simulink model "UNIFIER_dyn"  (R2023b)
settings: Solver=VariableStepAuto  StartTime=0.0  StopTime=10  RelTol=1e-3
InitFcn:
  | UNIFIER_LOAD
values from neighbouring files (symbols this model uses):
  b = 20.11467    [UNIFIER_LOAD.m]    (also in UNIFIER_LOAD.mat; UNIFIER_LOAD_ROM.m; UNIFIER_LOAD_ROM.mat)
  c = 1.43676    [UNIFIER_LOAD.m]    (also in UNIFIER_LOAD.mat; UNIFIER_LOAD_ROM.m; UNIFIER_LOAD_ROM.mat)
  dp_DEP =     [UNIFIER_LOAD.mat]    (also in UNIFIER_LOAD_ROM.mat)
  dp_FUSE_FIN =     [UNIFIER_LOAD.mat]
  dp_HTU =     [UNIFIER_LOAD.mat]    (also in UNIFIER_LOAD_ROM.mat)
  dp_VTAIL =     [UNIFIER_LOAD.mat]
  dp_VTAIL_INDUCED =     [UNIFIER_LOAD.mat]
  dp_WING_root =     [UNIFIER_LOAD.mat]
  dp_WING_tip =     [UNIFIER_LOAD.mat]
  I = [23600,     -0,  -1740 ... (first row only)    [UNIFIER_LOAD.m]    (also in UNIFIER_LOAD.mat = [23600  0  -1740; 0  89800  0; -1740  0  102000]; UNIFIER_LOAD_ROM.m = [23600,     -0,   -1740; UNIFIER_LOAD_ROM.mat = [23600  0  -1740; 0  89800  0; -1740  0  102000])
  m = 7057    [UNIFIER_LOAD.m]    (also in UNIFIER_LOAD.mat; UNIFIER_LOAD_ROM.m; UNIFIER_LOAD_ROM.mat)
  S = 29.98388    [UNIFIER_LOAD.m]    (also in UNIFIER_LOAD.mat; UNIFIER_LOAD_ROM.m; UNIFIER_LOAD_ROM.mat)
  vtail_nodes = [dp_VTAIL.Xs_LE;     dp_VTAIL.Ys_LE;     dp_VTAIL.Zs_LE]    [UNIFIER_LOAD.m]    (also in UNIFIER_LOAD.mat = [-16.4894695282 -2.83441376686 -2.73765826225 -16.1370849609)
  wing_nodes = [fliplr(dp_WING_tip.LE_Xs),fliplr(dp_WING_root.LE_Xs),dp_WING_root.LE_Xs,dp_WING_tip.LE_Xs;     fliplr(-dp_WING_tip.LE_Ys),fliplr(-dp_WING_root.LE_Ys),dp_WING_root.LE_Ys,dp_WING_tip.LE_Ys;     fliplr(dp_WING_tip.LE_Zs),fliplr(dp_WING_root.LE_Zs),dp_WING_root.LE_Zs,dp_WING_tip.LE_Zs]    [UNIFIER_LOAD.m]    (also in UNIFIER_LOAD.mat = [-7.70795631409 -9.67500019073 -0.98178178072 -7.66801691055)
  X = target.X    [OptimalTracking_UNIFIER_obj.m]
  xyz_cg = [-8.09,0,-0.2]    [UNIFIER_LOAD.m]    (also in UNIFIER_LOAD.mat = [-8.09 0 -0.2]; UNIFIER_LOAD_ROM.m; UNIFIER_LOAD_ROM.mat = [-8.09 0 -0.2])
  xyz_DEP = [ -6.9629998	-6.9210000	-6.8660002	-6.8099999	-6.7540002	-6.6999998	-6.6999998	-6.7540002	-6.8099999	-6.8660002	-6.9210000	-6.9629998 ... (first row only)    [UNIFIER_LOAD.m]    (also in UNIFIER_LOAD.mat = [-6.9629998 -10.05 -0.90899998 -6.921 -8.4499998 -0.792 -6.8; UNIFIER_LOAD_ROM.m; UNIFIER_LOAD_ROM.mat = [-6.9629998 -10.05 -0.90899998 -6.921 -8.4499998 -0.792 -6.8)
undefined symbols (not defined in the file or in its folder): OBM, U, unifier_obm
libraries: sharedutil x7, aerolibtransform2 x4, sharedtransform x2, aerolibatmos2 x1, matrix_library x1, shared6dofsys x1, shared6dof x1, simulink x1
(part 1 of 3)
settings Model: SimulationMode=rapid-accelerator  Creator=Reggie Johanes  LastModifiedBy=Reggie Johanes
settings DebuggingCC: ParameterPrecisionLossMsg=none

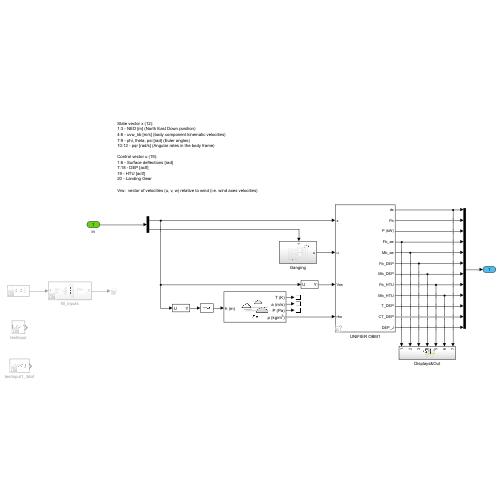
[thumbnail: Simulink's stored preview of the top-level diagram]
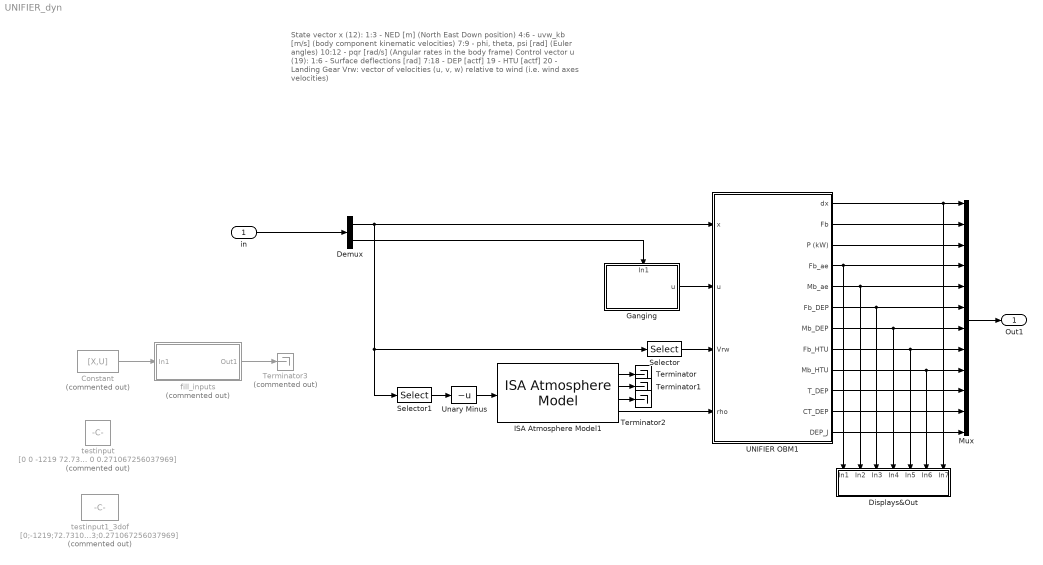
== system UNIFIER_dyn ==
  note: State vector x (12):
      | 1:3 - NED [m] (North East Down position)
      | 4:6 - uvw_kb [m/s] (body component kinematic velocities)
      | 7:9 - phi, theta, psi [rad] (Euler angles)
      | 10:12 - pqr [rad/s] (Angular rates in the body frame)
      |
      | Control vector u (19):
      | 1:6 - Surface deflections [rad]
      | 7:18 - DEP [actf]
      | 19 - HTU [actf]
      | 20 - Landing Gear
      |
      | Vrw:  vector of velocities (u, v, w) relative to wind (i.e. wind axes velocities)
  in : Inport
  Constant : Constant  Commented=on  Value=[X,U]
  Demux : Demux  Outputs=[12,7]
  Displays&Out : Subsystem
  Ganging : Subsystem
      settings: PortSchema="{\"entries\":[{\"content\":{\"sides\":[{\"content\":{},\"type\":\"ConnectorPlacement.EquallySpacedRectSide\",\"uuid\":\"ab643a29-1b81-4d77-b01e-60bacc52a34e\"},{\"content\":{\"connectorIds\":[\"Out1\"],\"side\":\"RIGHT\"},\"type\":\"ConnectorPlacement.EquallySpacedRectSide\",\"uuid\":\"168c35b5-3601-4e59-863f-07713e2152c6\"},{\"content\":{\"connectorIds\":[\"In1\"],\"side\":\"TOP\"},\"type\":\"ConnectorPlacement.EquallySpacedRectSide\",\"uuid\":\"1288536c-167d-4f59-8222-829bbd711e20\"}]},\"type\":\"ConnectorPlacement.EquallySpacedConnector\",\"uuid\":\"db641389-38bb-4549-8fb7-216d33e1be74\"}],\"packageUris\":[\"http://schema.mathworks.com/mf0/Connector/R2020b\"],\"version\":\"1.0\"}"
  ISA Atmosphere Model1 : aerolibatmos2/ISA Atmosphere Model  useExtended=off  action=Warning  custom=off  viscosityOut=off  g=9.80665  gamma=1.4  R=287.0531  L=0.0065  h_trop=11000  h_strat=20000  rho0=1.225  P0=101325  T0=288.15  h0=0
  Mux : Mux  Inputs=12
  Selector : Selector  InputPortWidth=12  IndexOptions=Index vector (dialog)  Indices=[4 5 6]  OutputSizes=1
  Selector1 : Selector  InputPortWidth=12  IndexOptions=Index vector (dialog)  Indices=[3]  OutputSizes=1
  Terminator : Terminator
  Terminator1 : Terminator
  Terminator2 : Terminator
  Terminator3 : Terminator  Commented=on
  UNIFIER OBM1 : Subsystem  AncestorBlock=unifier_obm/OBM
  Unary Minus : UnaryMinus
  fill_inputs : Subsystem  Commented=on
  testinput : Constant  Commented=on  Value=|
      | [0
      | 0
      | -1219
      | 72.7310470326144
      | 0
      | 1.14230710451874
      | 0
      | 0.0157060522826662
      | 0
      | 0
      | 0
      | 0
      | 0
      | 0
      | -0.0152983206921004
      | 0
      | 0.306978739246813
      | 0
      | 0.271067256037969]
  testinput1_3dof : Constant  Commented=on  Value=[0;-1219;72.731047032614440;1.142307104518741;0.015706052282666;0;-0.015298320692100;0;0.306978739246813;0.271067256037969]
  Out1 : Outport
  wires:
  Demux/1 -> Selector/1, Selector1/1, UNIFIER OBM1/1(x)
  Selector1/1 -> Unary Minus/1
  Unary Minus/1 -> ISA Atmosphere Model1/1
  ISA Atmosphere Model1/1 -> Terminator/1
  ISA Atmosphere Model1/2 -> Terminator1/1
  ISA Atmosphere Model1/3 -> Terminator2/1
  ISA Atmosphere Model1/4 -> UNIFIER OBM1/4(rho)
  Selector/1 -> UNIFIER OBM1/3(Vrw)
  Ganging/1(u) -> UNIFIER OBM1/2(u)
  Demux/2 -> Ganging/1(In1)
  UNIFIER OBM1/6(Fb_DEP) -> Mux/6, Displays&Out/3(In3)
  UNIFIER OBM1/4(Fb_ae) -> Mux/4, Displays&Out/1(In1)
  UNIFIER OBM1/7(Mb_DEP) -> Mux/7, Displays&Out/4(In4)
  UNIFIER OBM1/8(Fb_HTU) -> Mux/8, Displays&Out/5(In5)
  UNIFIER OBM1/11(CT_DEP) -> Mux/11
  UNIFIER OBM1/2(Fb) -> Mux/2
  UNIFIER OBM1/9(Mb_HTU) -> Mux/9, Displays&Out/6(In6)
  UNIFIER OBM1/3(P (kW)) -> Mux/3
  UNIFIER OBM1/10(T_DEP) -> Mux/10
  UNIFIER OBM1/1(dx) -> Displays&Out/7(In7), Mux/1
  Mux/1 -> Out1/1
  UNIFIER OBM1/12(DEP_J) -> Mux/12
  UNIFIER OBM1/5(Mb_ae) -> Mux/5, Displays&Out/2(In2)
  in/1 -> Demux/1
  Constant/1 -> fill_inputs/1(In1)
  fill_inputs/1(Out1) -> Terminator3/1

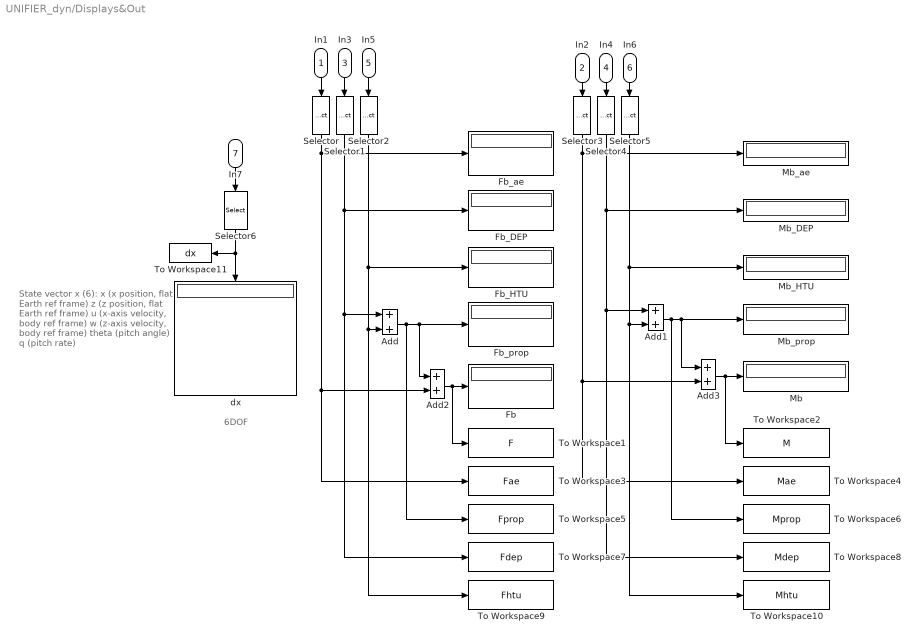
== system UNIFIER_dyn/Displays&Out ==
  note: State vector x (6):
      | x (x position, flat Earth ref frame)
      | z (z position, flat Earth ref frame)
      | u (x-axis velocity, body ref frame)
      | w (z-axis velocity, body ref frame)
      | theta (pitch angle)
      | q (pitch rate)
  note: 6DOF
  In1 : Inport
  In2 : Inport  Port=2
  In3 : Inport  Port=3
  In4 : Inport  Port=4
  In5 : Inport  Port=5
  In6 : Inport  Port=6
  In7 : Inport  Port=7
  Add{,1..3} (4 alike) : Sum
  Fb : Display
  Fb_DEP : Display
  Fb_HTU : Display
  Fb_ae : Display
  Fb_prop : Display
  Mb : Display
  Mb_DEP : Display
  Mb_HTU : Display
  Mb_ae : Display
  Mb_prop : Display
  Selector : Selector  InputPortWidth=3  IndexOptions=Index vector (dialog)  Indices=[1 3]  OutputSizes=1
  Selector1 : Selector  InputPortWidth=3  IndexOptions=Index vector (dialog)  Indices=[1 3]  OutputSizes=1
  Selector2 : Selector  InputPortWidth=3  IndexOptions=Index vector (dialog)  Indices=[1 3]  OutputSizes=1
  Selector3 : Selector  InputPortWidth=3  IndexOptions=Index vector (dialog)  Indices=[2]  OutputSizes=1
  Selector4 : Selector  InputPortWidth=3  IndexOptions=Index vector (dialog)  Indices=[2]  OutputSizes=1
  Selector5 : Selector  InputPortWidth=3  IndexOptions=Index vector (dialog)  Indices=[2]  OutputSizes=1
  Selector6 : Selector  InputPortWidth=12  IndexOptions=Index vector (dialog)  Indices=[1 3 4 6 8 11]  OutputSizes=1
  To Workspace1 : ToWorkspace  VariableName=F  SampleTime=-1
  To Workspace10 : ToWorkspace  VariableName=Mhtu  SampleTime=-1
  To Workspace11 : ToWorkspace  VariableName=dx  SampleTime=-1
  To Workspace2 : ToWorkspace  VariableName=M  SampleTime=-1
  To Workspace3 : ToWorkspace  VariableName=Fae  SampleTime=-1
  To Workspace4 : ToWorkspace  VariableName=Mae  SampleTime=-1
  To Workspace5 : ToWorkspace  VariableName=Fprop  SampleTime=-1
  To Workspace6 : ToWorkspace  VariableName=Mprop  SampleTime=-1
  To Workspace7 : ToWorkspace  VariableName=Fdep  SampleTime=-1
  To Workspace8 : ToWorkspace  VariableName=Mdep  SampleTime=-1
  To Workspace9 : ToWorkspace  VariableName=Fhtu  SampleTime=-1
  dx : Display
  wires:
  In5/1 -> Selector2/1
  Add1/1 -> Mb_prop/1, Add3/1, To Workspace6/1
  Add3/1 -> To Workspace2/1, Mb/1
  In3/1 -> Selector1/1
  Selector/1 -> To Workspace3/1, Add2/2, Fb_ae/1
  In4/1 -> Selector4/1
  Add/1 -> Add2/1, Fb_prop/1, To Workspace5/1
  In2/1 -> Selector3/1
  Add2/1 -> To Workspace1/1, Fb/1
  In6/1 -> Selector5/1
  In1/1 -> Selector/1
  Selector1/1 -> Fb_DEP/1, To Workspace7/1, Add/1
  Selector2/1 -> Add/2, To Workspace9/1, Fb_HTU/1
  Selector3/1 -> Mb_ae/1, To Workspace4/1, Add3/2
  Selector4/1 -> To Workspace8/1, Add1/1, Mb_DEP/1
  Selector5/1 -> Mb_HTU/1, To Workspace10/1, Add1/2
  Selector6/1 -> dx/1, To Workspace11/1
  In7/1 -> Selector6/1

== system UNIFIER_dyn/Ganging ==
  In1 : Inport
  Constant : Constant  Value=0
  Demux : Demux  Outputs=7
  For Each Subsystem : Subsystem  TreatAsAtomicUnit=on
  Mux : Mux  Inputs=2
  Mux1 : Mux  Inputs=2
  Mux2 : Mux  Inputs=2
  Mux3 : Mux
  Mux4 : Mux  Inputs=3
  Unary Minus : UnaryMinus
  V-tail mixing : Subsystem
  zeta : Constant  Value=[-1, -0.8, -0.4, -0.2, -0.1, 0, 0, 0.1, 0.2, 0.4, 0.8, 1]
  u : Outport
  wires:
  In1/1 -> Demux/1
  Mux3/1 -> u/1
  Demux/1 -> Mux/1, Unary Minus/1  "ail"
  Unary Minus/1 -> Mux/2
  V-tail mixing/1(rudL) -> Mux1/1
  V-tail mixing/2(rudR) -> Mux1/2
  Demux/4 -> Mux2/2, Mux2/1  "flap"
  Demux/7 -> Mux3/3  "u3"
  Mux/1 -> Mux4/1  "ail"
  Mux1/1 -> Mux4/2  "rud"
  Mux2/1 -> Mux4/3  "flap"
  Demux/5 -> For Each Subsystem/2(DEP_col)  "DEP_col"
  Demux/6 -> For Each Subsystem/3(DEP_slope)  "DEP_slp"
  For Each Subsystem/1(Out1) -> Mux3/2  "u2"
  Mux4/1 -> Mux3/1  "u1"
  Constant/1 -> Mux3/4  "u4"
  zeta/1 -> For Each Subsystem/1(zeta)
  Demux/2 -> V-tail mixing/1(rud)  "rud"
  Demux/3 -> V-tail mixing/2(elev)  "elev"

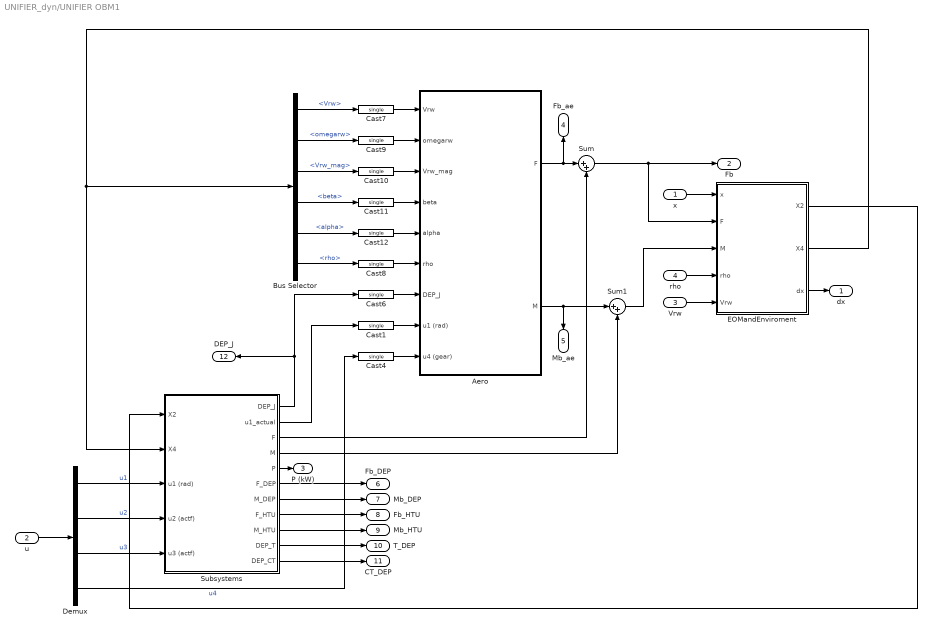
== system UNIFIER_dyn/UNIFIER OBM1 ==
  x : Inport
  u : Inport  Port=2
  Vrw : Inport  Port=3
  rho : Inport  Port=4
  Aero : Subsystem
  Bus Selector : BusSelector  OutputSignals=Vrw,omegarw,Vrw_mag,beta,alpha,rho
  Cast{1,4,6..12} (9 alike) : DataTypeConversion  OutDataTypeStr=single  SaturateOnIntegerOverflow=off  RndMeth=Floor
  Demux : Demux  Outputs=[6,12,1,1]
  EOMandEnviroment : Subsystem
  Subsystems : Subsystem
  Sum : Sum  Inputs=|++
  Sum1 : Sum  Inputs=|++
  dx : Outport
  Fb : Outport  Port=2
  P (kW) : Outport  Port=3
  Fb_ae : Outport  Port=4
  Mb_ae : Outport  Port=5
  Fb_DEP : Outport  Port=6
  Mb_DEP : Outport  Port=7
  Fb_HTU : Outport  Port=8
  Mb_HTU : Outport  Port=9
  T_DEP : Outport  Port=10
  CT_DEP : Outport  Port=11
  DEP_J : Outport  Port=12
  wires:
  Cast4/1 -> Aero/9(u4 (gear))
  Bus Selector/1 -> Cast7/1  "<Vrw>"
  Cast9/1 -> Aero/2(omegarw)
  EOMandEnviroment/2(X4) -> Bus Selector/1, Subsystems/2(X4)
  Cast10/1 -> Aero/3(Vrw_mag)
  Bus Selector/5 -> Cast12/1  "<alpha>"
  Cast7/1 -> Aero/1(Vrw)
  Cast8/1 -> Aero/6(rho)
  Bus Selector/3 -> Cast10/1  "<Vrw_mag>"
  Cast11/1 -> Aero/4(beta)
  Bus Selector/6 -> Cast8/1  "<rho>"
  Cast12/1 -> Aero/5(alpha)
  Bus Selector/2 -> Cast9/1  "<omegarw>"
  Bus Selector/4 -> Cast11/1  "<beta>"
  Vrw/1 -> EOMandEnviroment/5(Vrw)
  Subsystems/5(P) -> P (kW)/1
  Demux/4 -> Cast4/1  "u4"
  rho/1 -> EOMandEnviroment/4(rho)
  Demux/3 -> Subsystems/5(u3 (actf))  "u3"
  Demux/2 -> Subsystems/4(u2 (actf))  "u2"
  Demux/1 -> Subsystems/3(u1 (rad))  "u1"
  EOMandEnviroment/3(dx) -> dx/1
  x/1 -> EOMandEnviroment/1(x)
  u/1 -> Demux/1
  Aero/1(F) -> Fb_ae/1, Sum/1
  EOMandEnviroment/1(X2) -> Subsystems/1(X2)
  Aero/2(M) -> Sum1/1, Mb_ae/1
  Subsystems/1(DEP_J) -> DEP_J/1, Cast6/1
  Cast6/1 -> Aero/7(DEP_J)
  Sum/1 -> EOMandEnviroment/2(F), Fb/1
  Subsystems/2(u1_actual) -> Cast1/1
  Subsystems/3(F) -> Sum/2
  Subsystems/4(M) -> Sum1/2
  Cast1/1 -> Aero/8(u1 (rad))
  Sum1/1 -> EOMandEnviroment/3(M)
  Subsystems/6(F_DEP) -> Fb_DEP/1
  Subsystems/7(M_DEP) -> Mb_DEP/1
  Subsystems/8(F_HTU) -> Fb_HTU/1
  Subsystems/9(M_HTU) -> Mb_HTU/1
  Subsystems/11(DEP_CT) -> CT_DEP/1
  Subsystems/10(DEP_T) -> T_DEP/1

== system UNIFIER_dyn/fill_inputs ==
  note: 3DOF
      |
      | State vector x (6):
      | x (x position, flat Earth reference frame)
      | z (z position, flat Earth reference frame)
      | u (x-axis velocity, body reference frame)
      | w (z-axis velocity, body reference frame)
      | theta (pitch angle)
      | q (pitch rate)
      |
      | Control vector u (4):
      | dElev (elevator deflection)
      | dFlap (flap deflection)
      | DEP_col (DEP thrust level)
      | HTU (HTU thrust level)
  note: 6DOF
      |
      | State vector x (12):
      | 1:3 - NED [m] (North East Down position)
      | 4:6 - uvw_kb [m/s] (body component kinematic velocities)
      | 7:9 - phi, theta, psi [rad] (Euler angles)
      | 10:12 - pqr [rad/s] (Angular rates in the body frame)
      |
      | Control vector u (7) [GANGED]:
      | 1 - ail
      | 2 - rud
      | 3 - elev
      | 4 - flap
      | 5 - DEP_col
      | 6 - DEP_slope
      | 7 - HTU
  In1 : Inport
  Constant : Constant  Value=0
  Demux : Demux  Outputs=10
  Mux : Mux  Inputs=19
  Out1 : Outport
  wires:
  In1/1 -> Demux/1
  Demux/1 -> [x]  "x"
  Mux/1 -> Out1/1
  Demux/2 -> [z]  "z"
  Demux/10 -> [HTU]  "HTU"
  Demux/3 -> [u]  "u"
  Demux/4 -> [w]  "w"
  Demux/5 -> [theta]  "theta"
  Demux/6 -> [q]  "q"
  Demux/7 -> [dElev]  "dElev"
  Demux/8 -> [dFlap]  "dFlap"
  Demux/9 -> [DEP]  "DEP"
  [x] -> Mux/1
  [z] -> Mux/3
  [u] -> Mux/4
  [w] -> Mux/6
  [theta] -> Mux/8
  [q] -> Mux/11
  [dElev] -> Mux/15
  [dFlap] -> Mux/16
  [DEP] -> Mux/17
  [HTU] -> Mux/19
  Constant/1 -> Mux/2, Mux/18, Mux/14, Mux/13, Mux/12, Mux/10, Mux/9, Mux/7, Mux/5

== system UNIFIER_dyn/Ganging/For Each Subsystem ==
  zeta : Inport  Partition=on  PartitionDimension=1  PartitionWidth=1  PartitionOffset=0
  DEP_col : Inport  Port=2
  DEP_slope : Inport  Port=3
  Add : Sum
  Display : Display
  For Each : ForEach  DisableCoverage=on
  K_slope : Gain  Gain=0.785
  Product : Product
  Tan : Trigonometry  Operator=tan
  Out1 : Outport  ConcatenationDimension=1
  wires:
  DEP_slope/1 -> K_slope/1
  K_slope/1 -> Tan/1
  Tan/1 -> Product/1
  zeta/1 -> Product/2
  Product/1 -> Add/1
  DEP_col/1 -> Add/2
  Add/1 -> Display/1, Out1/1

== system UNIFIER_dyn/Ganging/V-tail mixing ==
  rud : Inport
  elev : Inport  Port=2
  Sum : Sum  Inputs=|++
  Sum1 : Sum  Inputs=|++
  Unary Minus1 : UnaryMinus
  rudL : Outport
  rudR : Outport  Port=2
  wires:
  Sum/1 -> rudL/1
  Sum1/1 -> rudR/1
  rud/1 -> Sum1/2, Unary Minus1/1
  Unary Minus1/1 -> Sum/2
  elev/1 -> Sum1/1, Sum/1

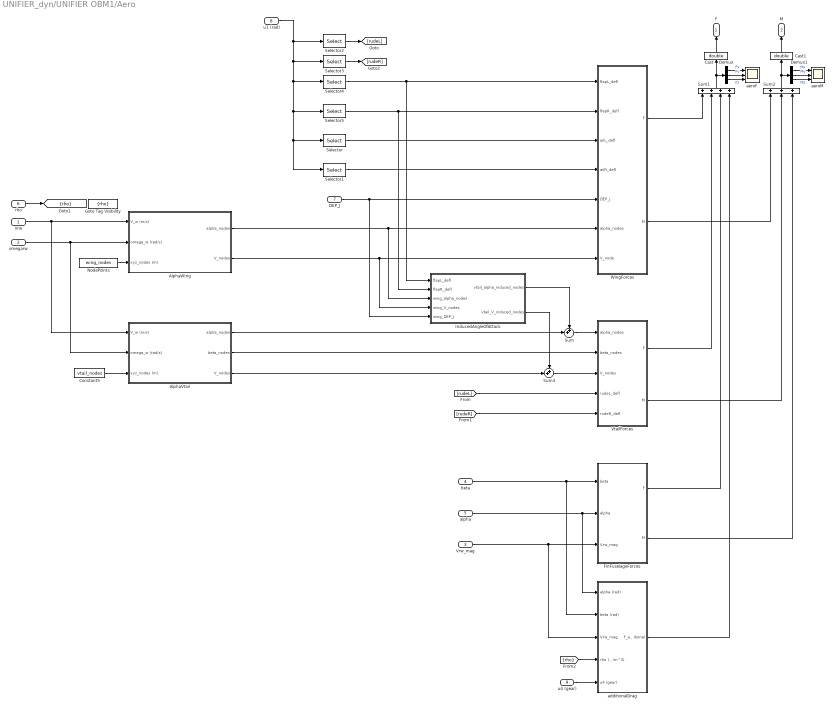
== system UNIFIER_dyn/UNIFIER OBM1/Aero ==
  Vrw : Inport  OutDataTypeStr=single  Unit=m/s  PortDimensions=3  LockScale=on
  omegarw : Inport  Port=2  OutDataTypeStr=single  Unit=rad/s  PortDimensions=3  LockScale=on
  Vrw_mag : Inport  Port=3  OutDataTypeStr=single
  beta : Inport  Port=4  OutDataTypeStr=single
  alpha : Inport  Port=5  OutDataTypeStr=single
  rho : Inport  Port=6  OutDataTypeStr=single  Unit=kg/m^3  PortDimensions=1  LockScale=on
  DEP_J : Inport  Port=7  OutDataTypeStr=single  PortDimensions=12  LockScale=on
  u1 (rad) : Inport  Port=8
  u4 (gear) : Inport  Port=9
  AlphaVtail : Subsystem  TreatAsAtomicUnit=on
  AlphaWIng : Subsystem  TreatAsAtomicUnit=on
  Cast : DataTypeConversion  OutDataTypeStr=double  SaturateOnIntegerOverflow=off  RndMeth=Floor
  Cast1 : DataTypeConversion  OutDataTypeStr=double  SaturateOnIntegerOverflow=off  RndMeth=Floor
  Constant5 : Constant  Value=vtail_nodes
  Demux : Demux  Outputs=3
  Demux1 : Demux  Outputs=3
  FinFuselageForces : Subsystem
  Goto Tag Visibility : GotoTagVisibility  GotoTag=rho
  InducedAngleOfAttack : Subsystem
  NodePoints : Constant  Value=wing_nodes
  Selector : Selector  InputPortWidth=6  IndexOptions=Index vector (dialog)  Indices=1  OutputSizes=1
  Selector1 : Selector  InputPortWidth=6  IndexOptions=Index vector (dialog)  Indices=2  OutputSizes=1
  Selector2 : Selector  InputPortWidth=6  IndexOptions=Index vector (dialog)  Indices=3  OutputSizes=1
  Selector3 : Selector  InputPortWidth=6  IndexOptions=Index vector (dialog)  Indices=4  OutputSizes=1
  Selector4 : Selector  InputPortWidth=6  IndexOptions=Index vector (dialog)  Indices=5  OutputSizes=1
  Selector5 : Selector  InputPortWidth=6  IndexOptions=Index vector (dialog)  Indices=6  OutputSizes=1
  Sum : Sum  Inputs=++|
  Sum1 : Sum  Inputs=++++
  Sum2 : Sum  Inputs=+++
  Sum3 : Sum  Inputs=++|
  VtailForces : Subsystem
  WingForces : Subsystem
  additionalDrag : Subsystem
  aeroF : Scope  NumInputPorts=3
  aeroM : Scope  NumInputPorts=3
  F : Outport  Unit=N  PortDimensions=3  LockScale=on
  M : Outport  Port=2  Unit=N*m  PortDimensions=3  LockScale=on
  tag scope: rho=scoped
  wires:
  u1 (rad)/1 -> Selector2/1, Selector3/1, Selector4/1, Selector5/1, Selector/1, Selector1/1
  u4 (gear)/1 -> additionalDrag/5(u4 (gear))
  additionalDrag/1(F_additional) -> Sum1/4
  [rho] -> additionalDrag/4(rho (kg/m^3))
  alpha/1 -> FinFuselageForces/2(alpha), additionalDrag/1(alpha (rad))
  AlphaWIng/1(alpha_nodes) -> InducedAngleOfAttack/3(wing_alpha_nodes), WingForces/6(alpha_nodes)
  Demux1/3 -> aeroM/3  "Mz"
  Demux1/1 -> aeroM/1  "Mx"
  Demux1/2 -> aeroM/2  "My"
  Sum2/1 -> Demux1/1, Cast1/1
  Demux/3 -> aeroF/3  "Fz"
  Demux/2 -> aeroF/2  "Fy"
  Demux/1 -> aeroF/1  "Fx"
  Selector3/1 -> [rudeR]
  Selector2/1 -> [rudeL]
  Selector5/1 -> InducedAngleOfAttack/2(flapR_defl), WingForces/2(flapR_defl)
  Selector4/1 -> InducedAngleOfAttack/1(flapL_defl), WingForces/1(flapL_defl)
  Selector1/1 -> WingForces/4(ailR_defl)
  Selector/1 -> WingForces/3(ailL_defl)
  FinFuselageForces/2(M) -> Sum2/3
  FinFuselageForces/1(F) -> Sum1/3
  beta/1 -> FinFuselageForces/1(beta), additionalDrag/2(beta (rad))
  Vrw_mag/1 -> FinFuselageForces/3(Vrw_mag), additionalDrag/3(Vrw_mag)
  Cast1/1 -> M/1
  Cast/1 -> F/1
  AlphaVtail/1(alpha_nodes) -> Sum/2
  Sum3/1 -> VtailForces/3(V_nodes)
  InducedAngleOfAttack/2(vtail_V_induced_nodes) -> Sum3/1
  InducedAngleOfAttack/1(vtail_alpha_induced_nodes) -> Sum/1
  AlphaVtail/3(V_nodes) -> Sum3/2
  Sum1/1 -> Cast/1, Demux/1
  VtailForces/2(M) -> Sum2/2
  WingForces/2(M) -> Sum2/1
  VtailForces/1(F) -> Sum1/2
  WingForces/1(F) -> Sum1/1
  [rudeR] -> VtailForces/5(rudeR_defl)
  [rudeL] -> VtailForces/4(rudeL_defl)
  AlphaVtail/2(beta_nodes) -> VtailForces/2(beta_nodes)
  rho/1 -> [rho]
  Sum/1 -> VtailForces/1(alpha_nodes)
  DEP_J/1 -> InducedAngleOfAttack/5(wing_DEP_J), WingForces/5(DEP_J)
  AlphaWIng/2(V_nodes) -> InducedAngleOfAttack/4(wing_V_nodes), WingForces/7(V_node)
  omegarw/1 -> AlphaWIng/2(omega_w (rad/s)), AlphaVtail/2(omega_w (rad/s))
  Vrw/1 -> AlphaWIng/1(V_w (m/s)), AlphaVtail/1(V_w (m/s))
  Constant5/1 -> AlphaVtail/3(xyz_nodes (m))
  NodePoints/1 -> AlphaWIng/3(xyz_nodes (m))

== system UNIFIER_dyn/UNIFIER OBM1/EOMandEnviroment ==
  note: State vector x (12):
      | 1:3 - NED [m] (North East Down position)
      | 4:6 - uvw_kb [m/s] (body component kinematic velocities)
      | 7:9 - phi, theta, psi [rad] (Euler angles)
      | 10:12 - pqr [rad/s] (Angular rates in the body frame)
  x : Inport
  F : Inport  Port=2
  M : Inport  Port=3
  rho : Inport  Port=4
  Vrw : Inport  Port=5
  Bus Creator : BusCreator  Inputs=8
  Conversion1 : Subsystem
  EOM : Subsystem  mask{mass=m, inertia=I}
      mask prompts: mass "Mass [kg]"; inertia "Inertia [kg/m^3]"
  Mux : Mux  Inputs=2
  Terminator : Terminator
  pqr : Selector  InputPortWidth=12  IndexOptions=Index vector (dialog)  Indices=10:12  OutputSizes=1
  X2 : Outport
  X4 : Outport  Port=2
  dx : Outport  Port=3
  wires:
  Vrw/1 -> Mux/1, Conversion1/1(Vrw), Bus Creator/2  "Vrw"
  Conversion1/2(Vrw_mag_eas) -> Bus Creator/4  "Vrw_mag_eas"
  EOM/2(Abe) -> Terminator/1
  Mux/1 -> X2/1
  rho/1 -> Bus Creator/8, Conversion1/2(rho)  "rho"
  EOM/1(dx) -> dx/1
  x/1 -> pqr/1, EOM/1(x)
  M/1 -> EOM/3(M)
  F/1 -> EOM/2(F)
  EOM/3(DCMbe) -> Bus Creator/1  "DCMbe"
  pqr/1 -> Mux/2, Bus Creator/7  "omegarw"
  Conversion1/1(Vrw_mag) -> Bus Creator/3  "Vrw_mag"
  Conversion1/4(beta) -> Bus Creator/6  "beta"
  Bus Creator/1 -> X4/1
  Conversion1/3(alpha) -> Bus Creator/5  "alpha"

== system UNIFIER_dyn/UNIFIER OBM1/Subsystems ==
  X2 : Inport
  X4 : Inport  Port=2
  u1 (rad) : Inport  Port=3
  u2 (actf) : Inport  Port=4
  u3 (actf) : Inport  Port=5
  Actuators : Subsystem
  DEP1 : Subsystem
  Gravity : Subsystem
  HTU : Subsystem
  Sum : Sum  Inputs=+++
  Sum1 : Sum
  Sum2 : Sum  Inputs=|++
  DEP_J : Outport
  u1_actual : Outport  Port=2
  F : Outport  Port=3
  M : Outport  Port=4
  P : Outport  Port=5
  F_DEP : Outport  Port=6
  M_DEP : Outport  Port=7
  F_HTU : Outport  Port=8
  M_HTU : Outport  Port=9
  DEP_T : Outport  Port=10
  DEP_CT : Outport  Port=11
  wires:
  Sum2/1 -> P/1
  HTU/3(P (kW)) -> Sum2/2
  DEP1/4(P (kW)) -> Sum2/1
  u2 (actf)/1 -> DEP1/3(u2 (actf))
  u3 (actf)/1 -> HTU/1(u3 (actf))
  Actuators/1(u1_actual) -> u1_actual/1
  u1 (rad)/1 -> Actuators/1(u1)
  DEP1/3(M) -> Sum1/1, M_DEP/1
  DEP1/2(F) -> Sum/1, F_DEP/1
  HTU/2(M (Nm)) -> M_HTU/1, Sum1/2
  Sum1/1 -> M/1
  HTU/1(F (N)) -> F_HTU/1, Sum/3
  Gravity/1(F) -> Sum/2
  Sum/1 -> F/1
  DEP1/1(DEP_J) -> DEP_J/1
  X4/1 -> DEP1/2(X4), Gravity/1(X4), HTU/2(X4)
  X2/1 -> DEP1/1(X2)
  DEP1/5(DEP_T) -> DEP_T/1
  DEP1/6(DEP_CT) -> DEP_CT/1

== system UNIFIER_dyn/UNIFIER OBM1/Aero/AlphaVtail ==
  V_w (m/s) : Inport
  omega_w (rad/s) : Inport  Port=2
  xyz_nodes (m) : Inport  Port=3  Partition=on  PartitionDimension=2  PartitionWidth=1  PartitionOffset=0
  3x3 Cross Product : sharedutil/3x3 Cross Product  aMode=aMode
  Asin : Trigonometry  Operator=asin
  Atan : Trigonometry  Operator=atan
  Cast : DataTypeConversion  OutDataTypeStr=single  SaturateOnIntegerOverflow=off  RndMeth=Floor
  Constant : Constant  Value=xyz_cg
  Constant1 : Constant  Value=eps  OutDataTypeStr=single
  Demux : Demux  Outputs=3
  Divide : Product  Inputs=*/
  Divide1 : Product  Inputs=*/
  For Each : ForEach  DisableCoverage=on  SpecifiedNumIters=16
  Mux : Mux  Inputs=3
  Sum : Sum  Inputs=+-
  Sum1 : Sum  Inputs=++|
  Sum2 : Sum  Inputs=|++
  Sum3 : Sum  Inputs=|++
  V_inf : Fcn  Expr=sqrt(u(1)^2+u(2)^2+u(3)^2)
  alpha_nodes : Outport  ConcatenationDimension=2
  beta_nodes : Outport  Port=2  ConcatenationDimension=2
  V_nodes : Outport  Port=3  ConcatenationDimension=2
  wires:
  Cast/1 -> Sum/1
  Sum3/1 -> Divide1/2, V_nodes/1
  V_inf/1 -> Sum3/1
  Asin/1 -> beta_nodes/1  "beta"
  Mux/1 -> V_inf/1
  Demux/2 -> Divide1/1, Mux/2
  Divide1/1 -> Asin/1
  Constant1/1 -> Sum2/2, Sum3/2
  Sum2/1 -> Divide/2
  Atan/1 -> alpha_nodes/1
  Divide/1 -> Atan/1
  Demux/3 -> Divide/1, Mux/3  "w"
  Demux/1 -> Mux/1, Sum2/1  "u"
  Sum1/1 -> Demux/1
  V_w (m/s)/1 -> Sum1/2
  omega_w (rad/s)/1 -> 3x3 Cross Product/2
  xyz_nodes (m)/1 -> Sum/2
  Constant/1 -> Cast/1
  Sum/1 -> 3x3 Cross Product/1
  3x3 Cross Product/1 -> Sum1/1

== system UNIFIER_dyn/UNIFIER OBM1/Aero/AlphaWIng ==
  V_w (m/s) : Inport
  omega_w (rad/s) : Inport  Port=2
  xyz_nodes (m) : Inport  Port=3  Partition=on  PartitionDimension=2  PartitionWidth=1  PartitionOffset=0
  Cast : DataTypeConversion  OutDataTypeStr=single  SaturateOnIntegerOverflow=off  RndMeth=Floor
  ComputeAlphaBetaV : Subsystem
  Constant : Constant  Value=xyz_cg
  Cross Product : matrix_library/Cross Product
  For Each : ForEach  DisableCoverage=on  SpecifiedNumIters=14
  Sum : Sum  Inputs=+-
  Sum1 : Sum  Inputs=++|
  Terminator : Terminator
  alpha_nodes : Outport  ConcatenationDimension=2
  V_nodes : Outport  Port=2  ConcatenationDimension=2
  wires:
  ComputeAlphaBetaV/1(alpha_nodes) -> alpha_nodes/1
  ComputeAlphaBetaV/2(beta_nodes) -> Terminator/1
  ComputeAlphaBetaV/3(V_nodes) -> V_nodes/1
  Sum1/1 -> ComputeAlphaBetaV/1(V_w_local)
  Cast/1 -> Sum/1
  V_w (m/s)/1 -> Sum1/2
  omega_w (rad/s)/1 -> Cross Product/2
  xyz_nodes (m)/1 -> Sum/2
  Constant/1 -> Cast/1
  Sum/1 -> Cross Product/1
  Cross Product/1 -> Sum1/1

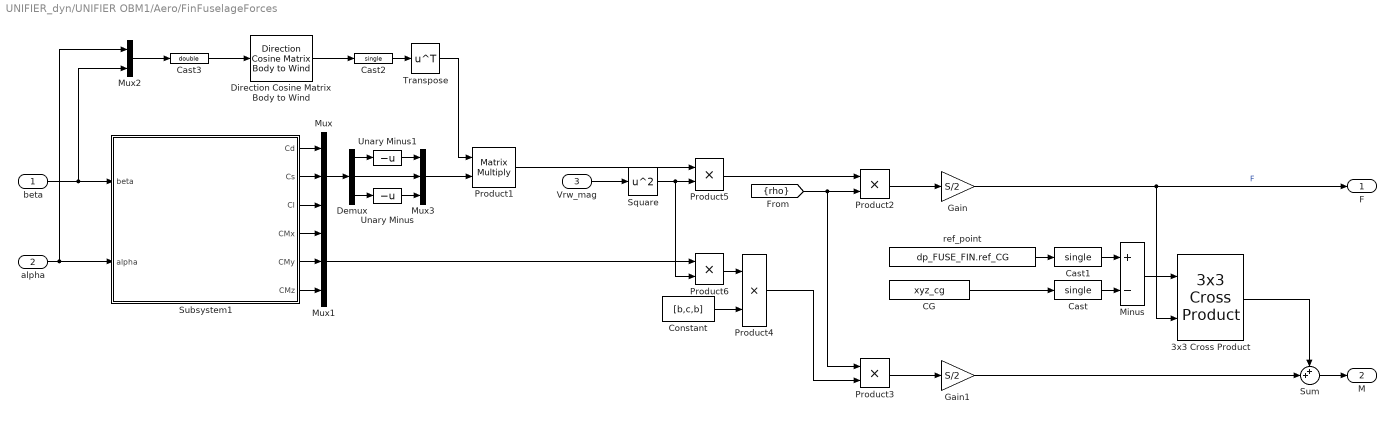
== system UNIFIER_dyn/UNIFIER OBM1/Aero/FinFuselageForces ==
  beta : Inport
  alpha : Inport  Port=2
  Vrw_mag : Inport  Port=3  OutDataTypeStr=single
  3x3 Cross Product : sharedutil/3x3 Cross Product  aMode=aMode
  CG : Constant  Value=xyz_cg
  Cast : DataTypeConversion  OutDataTypeStr=single  SaturateOnIntegerOverflow=off  RndMeth=Floor
  Cast1 : DataTypeConversion  OutDataTypeStr=single  SaturateOnIntegerOverflow=off  RndMeth=Floor
  Cast2 : DataTypeConversion  OutDataTypeStr=single  SaturateOnIntegerOverflow=off  RndMeth=Floor
  Cast3 : DataTypeConversion  OutDataTypeStr=double  SaturateOnIntegerOverflow=off  RndMeth=Floor
  Constant : Constant  Value=[b,c,b]
  Demux : Demux  Outputs=3
  Direction Cosine Matrix Body to Wind : aerolibtransform2/Direction Cosine Matrix Body to Wind
  Gain : Gain  Gain=S/2
  Gain1 : Gain  Gain=S/2
  Minus : Sum  Inputs=+-
  Mux : Mux  Inputs=3
  Mux1 : Mux  Inputs=3
  Mux2 : Mux  Inputs=2
  Mux3 : Mux  Inputs=3
  Product1 : Product  Multiplication=Matrix(*)
  Product{2..6} (5 alike) : Product
  Square : Math  Operator=square
  Subsystem1 : Subsystem
  Sum : Sum  Inputs=++|
  Transpose : Math  Operator=transpose
  Unary Minus : UnaryMinus
  Unary Minus1 : UnaryMinus
  ref_point : Constant  Value=dp_FUSE_FIN.ref_CG
  F : Outport
  M : Outport  Port=2
  wires:
  Product2/1 -> Gain/1
  Product4/1 -> Product3/2
  Gain1/1 -> Sum/2
  [rho] -> Product2/2, Product3/1
  Constant/1 -> Product4/2
  Gain/1 -> F/1, 3x3 Cross Product/2  "F"
  Product3/1 -> Gain1/1
  Subsystem1/1(Cd) -> Mux/1
  Subsystem1/2(Cs) -> Mux/2
  Subsystem1/3(Cl) -> Mux/3
  Subsystem1/4(CMx) -> Mux1/1
  Subsystem1/5(CMy) -> Mux1/2
  Subsystem1/6(CMz) -> Mux1/3
  3x3 Cross Product/1 -> Sum/1
  ref_point/1 -> Cast1/1
  Cast/1 -> Minus/2
  Minus/1 -> 3x3 Cross Product/1
  CG/1 -> Cast/1
  Cast1/1 -> Minus/1
  beta/1 -> Mux2/2, Subsystem1/1(beta)
  alpha/1 -> Mux2/1, Subsystem1/2(alpha)
  Sum/1 -> M/1
  Mux2/1 -> Cast3/1
  Transpose/1 -> Product1/1
  Direction Cosine Matrix Body to Wind/1 -> Cast2/1
  Cast3/1 -> Direction Cosine Matrix Body to Wind/1
  Cast2/1 -> Transpose/1
  Demux/1 -> Unary Minus1/1
  Demux/2 -> Mux3/2
  Demux/3 -> Unary Minus/1
  Mux3/1 -> Product1/2
  Unary Minus/1 -> Mux3/3
  Unary Minus1/1 -> Mux3/1
  Square/1 -> Product6/2, Product5/2
  Product1/1 -> Product5/1
  Vrw_mag/1 -> Square/1
  Product5/1 -> Product2/1
  Mux1/1 -> Product6/1
  Product6/1 -> Product4/1
  Mux/1 -> Demux/1

== system UNIFIER_dyn/UNIFIER OBM1/Aero/InducedAngleOfAttack ==
  flapL_defl : Inport
  flapR_defl : Inport  Port=2
  wing_alpha_nodes : Inport  Port=3  PortDimensions=14
  wing_V_nodes : Inport  Port=4  PortDimensions=14
  wing_DEP_J : Inport  Port=5  PortDimensions=12
  1-D Lookup Table : Lookup_n-D  NumberOfTableDimensions=1  BreakpointsForDimension1=wing_nodes(2,5:10)  BeginIndexSearchUsingPreviousIndexResult=on  TableSource=Input port  Table=tanh([-5:5])  ExtrapMethod=Clip  InternalRulePriority=Speed  RndMeth=Simplest
      settings: InputPortMap=u0,p221
  1-D Lookup Table1 : Lookup_n-D  NumberOfTableDimensions=1  BreakpointsForDimension1=wing_nodes(2,5:10)  BeginIndexSearchUsingPreviousIndexResult=on  TableSource=Input port  Table=tanh([-5:5])  ExtrapMethod=Clip  InternalRulePriority=Speed  RndMeth=Simplest
      settings: InputPortMap=u0,p221
  1-D Lookup Table2 : Lookup_n-D  NumberOfTableDimensions=1  BreakpointsForDimension1=wing_nodes(2,5:10)  BeginIndexSearchUsingPreviousIndexResult=on  TableSource=Input port  Table=tanh([-5:5])  ExtrapMethod=Clip  InternalRulePriority=Speed  RndMeth=Simplest
      settings: InputPortMap=u0,p221
  Constant : Constant  Value=ones(1,8)
  Constant1 : Constant  Value=ones(1,8)
  Constant7 : Constant  Value=vtail_nodes(2,:)
  Mux : Mux  Inputs=2
  Product : Product
  Product1 : Product
  Selector : Selector  InputPortWidth=14  IndexOptions=Index vector (dialog)  Indices=[5:10]  OutputSizes=1
  Selector1 : Selector  InputPortWidth=14  IndexOptions=Index vector (dialog)  Indices=[5:10]  OutputSizes=1
  Selector2 : Selector  InputPortWidth=12  IndexOptions=Index vector (dialog)  Indices=[4:9]  OutputSizes=1
  V_induced : Interpolation_n-D  NumberOfTableDimensions=5  Table=dp_VTAIL_INDUCED.V_induced  NumSelectionDims=1  InternalRulePriority=Speed  TableDataTypeStr=Inherit: Inherit from 'Table data'
      settings: InputPortMap=u0,u1,u2,u3,u4,u5,u6,u7,u8
  alpha_induced : Interpolation_n-D  NumberOfTableDimensions=5  Table=dp_VTAIL_INDUCED.alpha_induced  NumSelectionDims=1  InternalRulePriority=Speed  TableDataTypeStr=Inherit: Inherit from 'Table data'
      settings: InputPortMap=u0,u1,u2,u3,u4,u5,u6,u7,u8
  preLook : Subsystem
  vtail_alpha_induced_nodes : Outport  PortDimensions=16
  vtail_V_induced_nodes : Outport  Port=2  PortDimensions=16
  wires:
  Selector2/1 -> 1-D Lookup Table2/2
  Selector1/1 -> 1-D Lookup Table1/2
  Selector/1 -> 1-D Lookup Table/2
  alpha_induced/1 -> vtail_alpha_induced_nodes/1
  V_induced/1 -> vtail_V_induced_nodes/1
  Mux/1 -> preLook/1(wing_flap_defl)
  Product1/1 -> Mux/2
  Product/1 -> Mux/1
  flapR_defl/1 -> Product1/2
  Constant1/1 -> Product1/1
  Constant/1 -> Product/1
  flapL_defl/1 -> Product/2
  wing_DEP_J/1 -> Selector2/1
  preLook/9(Out5) -> V_induced/9, alpha_induced/9
  preLook/8(Out7) -> V_induced/8, alpha_induced/8
  preLook/7(Out6) -> V_induced/7, alpha_induced/7
  preLook/6(Out4) -> V_induced/6, alpha_induced/6
  preLook/5(Out3) -> V_induced/5, alpha_induced/5
  preLook/4(Out9) -> V_induced/4, alpha_induced/4
  preLook/3(Out8) -> V_induced/3, alpha_induced/3
  preLook/2(Out2) -> V_induced/2, alpha_induced/2
  preLook/1(Out1) -> V_induced/1, alpha_induced/1
  wing_alpha_nodes/1 -> Selector/1
  wing_V_nodes/1 -> Selector1/1
  Constant7/1 -> 1-D Lookup Table1/1, 1-D Lookup Table2/1, 1-D Lookup Table/1
  1-D Lookup Table/1 -> preLook/2(wing_alphas)
  1-D Lookup Table2/1 -> preLook/4(wing_DEP_J)
  1-D Lookup Table1/1 -> preLook/3(wing_V_inf)

== system UNIFIER_dyn/UNIFIER OBM1/Aero/VtailForces ==
  alpha_nodes : Inport  PortDimensions=16
  beta_nodes : Inport  Port=2  PortDimensions=16
  V_nodes : Inport  Port=3  PortDimensions=16
  rudeL_defl : Inport  Port=4
  rudeR_defl : Inport  Port=5
  Constant : Constant  Value=ones(1,8)
  Constant1 : Constant  Value=ones(1,8)
  Matrix Concatenate1 : Concatenate  NumInputs=3  Mode=Multidimensional array  ConcatenateDimension=2
  Matrix Concatenate2 : Concatenate  NumInputs=3  Mode=Multidimensional array  ConcatenateDimension=2
  Mux : Mux  Inputs=2
  Product : Product
  Product1 : Product
  Reshape : Reshape
  Reshape1 : Reshape
  Subsystem : Subsystem
  Transpose : Math  Operator=transpose
  Transpose1 : Math  Operator=transpose
  VtailForces : Subsystem
  F : Outport
  M : Outport  Port=2
  wires:
  Reshape1/1 -> F/1
  Reshape/1 -> M/1
  V_nodes/1 -> Subsystem/1(V_nodes)
  VtailForces/3(Cz) -> Matrix Concatenate1/3  "CFz"
  Subsystem/1(F) -> Reshape1/1
  Matrix Concatenate1/1 -> Transpose/1
  VtailForces/1(Cx) -> Matrix Concatenate1/1  "CFx"
  VtailForces/5(CMy) -> Matrix Concatenate2/2  "CMy"
  VtailForces/2(Cy) -> Matrix Concatenate1/2  "CFy"
  Transpose1/1 -> Subsystem/3(M_matrix)
  Transpose/1 -> Subsystem/2(F_matrix)
  Subsystem/2(M) -> Reshape/1
  Matrix Concatenate2/1 -> Transpose1/1
  VtailForces/6(CMz) -> Matrix Concatenate2/3  "CMz"
  VtailForces/4(CMx) -> Matrix Concatenate2/1  "CMx"
  rudeR_defl/1 -> Product1/2
  rudeL_defl/1 -> Product/2
  Constant/1 -> Product/1
  Constant1/1 -> Product1/1
  Mux/1 -> VtailForces/1(rude_defl_nodes)
  Product1/1 -> Mux/2
  Product/1 -> Mux/1
  beta_nodes/1 -> VtailForces/3(beta_nodes)
  alpha_nodes/1 -> VtailForces/2(alpha_nodes)

== system UNIFIER_dyn/UNIFIER OBM1/Aero/WingForces ==
  flapL_defl : Inport
  flapR_defl : Inport  Port=2
  ailL_defl : Inport  Port=3
  ailR_defl : Inport  Port=4
  DEP_J : Inport  Port=5  PortDimensions=12
  alpha_nodes : Inport  Port=6  PortDimensions=14
  V_node : Inport  Port=7  PortDimensions=14
  Demux : Demux  Outputs=3
  Demux1 : Demux  Outputs=3
  Left : Subsystem
  Mux : Mux  Inputs=3
  Mux1 : Mux  Inputs=3
  Reshape : Reshape
  Reshape1 : Reshape
  Right : Subsystem
  Subsystem : Subsystem
  Sum : Sum  Inputs=|++
  Sum1 : Sum  Inputs=|++
  Unary Minus : UnaryMinus
  Unary Minus1 : UnaryMinus
  Unary Minus2 : UnaryMinus
  F : Outport
  M : Outport  Port=2
  wires:
  Reshape1/1 -> Sum1/2
  Reshape/1 -> Sum/2
  Subsystem/4(DEP_J_Right) -> Right/3(DEP_J)
  Subsystem/6(V_nodes_Right) -> Right/5(V_node)
  Subsystem/5(alpha_nodes_Right) -> Right/4(alpha)
  Right/2(M) -> Reshape1/1
  Right/1(F) -> Reshape/1
  Sum1/1 -> M/1
  Mux/1 -> Sum1/1
  Sum/1 -> F/1
  Mux1/1 -> Sum/1
  Demux/3 -> Mux1/3
  Demux/1 -> Mux1/1
  Unary Minus/1 -> Mux1/2
  Unary Minus2/1 -> Mux/3
  Unary Minus1/1 -> Mux/1
  Demux1/2 -> Mux/2
  Demux1/3 -> Unary Minus2/1
  Demux1/1 -> Unary Minus1/1
  Demux/2 -> Unary Minus/1
  Left/2(M) -> Demux1/1
  Left/1(F) -> Demux/1
  Subsystem/3(V_nodes_Left) -> Left/5(V_node)
  Subsystem/2(alpha_nodes_Left) -> Left/4(alpha)
  Subsystem/1(DEP_J_Left) -> Left/3(DEP_J)
  V_node/1 -> Subsystem/3(V_nodes)
  alpha_nodes/1 -> Subsystem/2(alpha_nodes)
  flapR_defl/1 -> Right/1(flap_defl)
  DEP_J/1 -> Subsystem/1(DEP_J)
  ailR_defl/1 -> Right/2(aile_defl)
  flapL_defl/1 -> Left/1(flap_defl)
  ailL_defl/1 -> Left/2(aile_defl)

== system UNIFIER_dyn/UNIFIER OBM1/Aero/additionalDrag ==
  note: Wing mounted nacelles:
      | (Estimate using OpenVSP - Jenkinson Wing Mounted Nacelle)
      | =6*0.00043=0.00258
      | + cooling drag of 0.015
  note: Landing gear drag:
      | Loftin Jr, L. K. (1980). Subsonic aircraft: Evolution and the matching of size to performance (No. L-13367).
  alpha (rad) : Inport
  beta (rad) : Inport  Port=2
  Vrw_mag : Inport  Port=3
  rho (kg/m^3) : Inport  Port=4
  u4 (gear) : Inport  Port=5
  Cast : DataTypeConversion  OutDataTypeStr=single  SaturateOnIntegerOverflow=off  RndMeth=Floor
  Cast1 : DataTypeConversion  OutDataTypeStr=single  SaturateOnIntegerOverflow=off  RndMeth=Floor
  Cast2 : DataTypeConversion  OutDataTypeStr=double  SaturateOnIntegerOverflow=off  RndMeth=Floor
  Constant1 : Constant  Value=0  OutDataTypeStr=single
  Direction Cosine Matrix Body to Wind : aerolibtransform2/Direction Cosine Matrix Body to Wind
  Gain : Gain  Gain=S/2
  Math Function : Math  Operator=square
  Mux : Mux  Inputs=2
  Mux1 : Mux  Inputs=3
  Product : Product  OutDataTypeStr=single
  Product1 : Product  Multiplication=Matrix(*)
  Product2 : Product
  Product3 : Product
  Sum : Sum  Inputs=|++
  Transpose : Math  Operator=transpose
  Unary Minus : UnaryMinus
  extra_drag : Constant  Value=0.00258+0.015  OutDataTypeStr=single
  gear_drag : Constant  Value=0.015  OutDataTypeStr=single
  F_additional : Outport
  wires:
  Product3/1 -> Sum/2
  Sum/1 -> Product2/1
  gear_drag/1 -> Product3/1
  u4 (gear)/1 -> Product3/2
  Cast2/1 -> Direction Cosine Matrix Body to Wind/1
  Cast1/1 -> Transpose/1
  Cast/1 -> F_additional/1
  Product1/1 -> Cast/1
  Constant1/1 -> Mux1/3, Mux1/2
  Mux1/1 -> Product1/2
  Transpose/1 -> Product1/1
  Unary Minus/1 -> Mux1/1
  beta (rad)/1 -> Mux/2
  Mux/1 -> Cast2/1
  Direction Cosine Matrix Body to Wind/1 -> Cast1/1
  rho (kg/m^3)/1 -> Product2/2
  Vrw_mag/1 -> Math Function/1
  extra_drag/1 -> Sum/1
  Product2/1 -> Gain/1
  Gain/1 -> Product/1
  Product/1 -> Unary Minus/1
  Math Function/1 -> Product/2
  alpha (rad)/1 -> Mux/1

== system UNIFIER_dyn/UNIFIER OBM1/EOMandEnviroment/Conversion1 ==
  Vrw : Inport
  rho : Inport  Port=2
  Add : Sum
  Constant1 : Constant  Value=eps
  Demux3 : Demux  Outputs=3
  Divide1 : Product  Inputs=*/
  Dot Product : DotProduct  OutDataTypeStr=Inherit: Inherit via internal rule
  Gain : Gain  Gain=1/1.225
  Product : Product
  Sqrt : Sqrt
  Sqrt1 : Sqrt
  Trigonometric Function : Trigonometry  Operator=atan2
  Trigonometric Function1 : Trigonometry  Operator=asin
  Vrw_mag : Outport
  Vrw_mag_eas : Outport  Port=2
  alpha : Outport  Port=3
  beta : Outport  Port=4
  wires:
  Add/1 -> Divide1/2, Product/1, Vrw_mag/1
  Product/1 -> Vrw_mag_eas/1
  Sqrt1/1 -> Product/2
  Gain/1 -> Sqrt1/1
  rho/1 -> Gain/1
  Trigonometric Function/1 -> alpha/1  "alpha"
  Trigonometric Function1/1 -> beta/1  "beta"
  Demux3/1 -> Trigonometric Function/2
  Dot Product/1 -> Sqrt/1
  Demux3/3 -> Trigonometric Function/1
  Vrw/1 -> Demux3/1, Dot Product/2, Dot Product/1  "V_w"
  Divide1/1 -> Trigonometric Function1/1
  Sqrt/1 -> Add/1
  Constant1/1 -> Add/2
  Demux3/2 -> Divide1/1

== system UNIFIER_dyn/UNIFIER OBM1/EOMandEnviroment/EOM ==
  note: DCM, NED_dot
  note: pqr_dot
  note: Euler_dot
  note: Linear acceleration
  x : Inport
  F : Inport  Port=2
  M : Inport  Port=3
  Calculate omega_dot : shared6dofsys/Calculate omega_dot  aMode=aMode
  Constant : Constant  Value=mass
  Constant1 : Constant  Value=inertia
  Constant2 : Constant  Value=zeros(3)
  Demux : Demux  Outputs=[3, 3, 3, 3]
  Mux6 : Mux
  Product : Product  Inputs=*/  SaturateOnIntegerOverflow=on  OutDataTypeStr=Inherit: Same as first input
  Rotation Angles to Direction Cosine Matrix : sharedtransform/Rotation Angles to Direction Cosine Matrix  rotationOrder=ZYX  aMode=aMode
  Selector : Selector  InputPortWidth=3  IndexOptions=Index vector (dialog)  Indices=[3 2 1]  OutputSizes=1
  Subsystem : Subsystem
  Sum : Sum  Inputs=|++  SaturateOnIntegerOverflow=on
  Terminator : Terminator
  Transpose : Math  Operator=transpose  SignedPower=on
  Vbxw : sharedutil/3x3 Cross Product  aMode=aMode
  Vector Concatenate : Concatenate  Mode=Multidimensional array
  "transform to Inertial axes " : shared6dof/6DOF (Euler Angles)/transform to Inertial axes   SystemSampleTime=-1  VariantActivationTime=update diagram  AllowFlexibleInterface=on  Latency=0  AutoFrameSizeCalculation=off
  dx : Outport
  Abe : Outport  Port=2
  DCMbe : Outport  Port=3
  wires:
  Demux/1 -> Terminator/1  "NED"
  Demux/2 -> "transform to Inertial axes "/1, Vbxw/1  "uvw_kb"
  Constant2/1 -> Vector Concatenate/2
  Calculate omega_dot/1 -> Mux6/4
  Demux/3 -> Selector/1, Subsystem/2(phi theta psi)  "phithepsi"
  Selector/1 -> Rotation Angles to Direction Cosine Matrix/1
  Constant/1 -> Product/2
  Rotation Angles to Direction Cosine Matrix/1 -> Transpose/1, DCMbe/1  "DCMbe"
  Demux/4 -> Vbxw/2, Calculate omega_dot/1, Subsystem/1(p q r)  "pqr"
  Mux6/1 -> dx/1
  Subsystem/1(phidot thetadot psidot) -> Mux6/3
  Constant1/1 -> Vector Concatenate/1
  M/1 -> Calculate omega_dot/3
  Vector Concatenate/1 -> Calculate omega_dot/2
  Product/1 -> Sum/1, Abe/1  "Abe"
  Sum/1 -> Mux6/2  "Abb"
  "transform to Inertial axes "/1 -> Mux6/1  "Ve"
  Vbxw/1 -> Sum/2
  F/1 -> Product/1
  Transpose/1 -> "transform to Inertial axes "/2
  x/1 -> Demux/1

== system UNIFIER_dyn/UNIFIER OBM1/Subsystems/Actuators ==
  u1 : Inport
  Demux : Demux  Outputs=6
  Mux : Mux  Inputs=6
  Saturation : Saturate  UpperLimit=deg2rad(25)  LowerLimit=deg2rad(-25)
  Saturation1 : Saturate  UpperLimit=deg2rad(25)  LowerLimit=deg2rad(-25)
  Saturation2 : Saturate  UpperLimit=deg2rad(30)  LowerLimit=deg2rad(-30)
  Saturation3 : Saturate  UpperLimit=deg2rad(30)  LowerLimit=deg2rad(-30)
  Saturation4 : Saturate  UpperLimit=deg2rad(25)  LowerLimit=0
  Saturation6 : Saturate  UpperLimit=deg2rad(25)  LowerLimit=0
  u1_actual : Outport
  wires:
  Saturation4/1 -> Mux/6
  Saturation6/1 -> Mux/5
  Demux/6 -> Saturation4/1
  Demux/5 -> Saturation6/1
  Mux/1 -> u1_actual/1
  Saturation/1 -> Mux/1
  Saturation1/1 -> Mux/2
  Saturation2/1 -> Mux/3
  Saturation3/1 -> Mux/4
  Demux/4 -> Saturation3/1
  Demux/3 -> Saturation2/1
  Demux/2 -> Saturation1/1
  Demux/1 -> Saturation/1
  u1/1 -> Demux/1

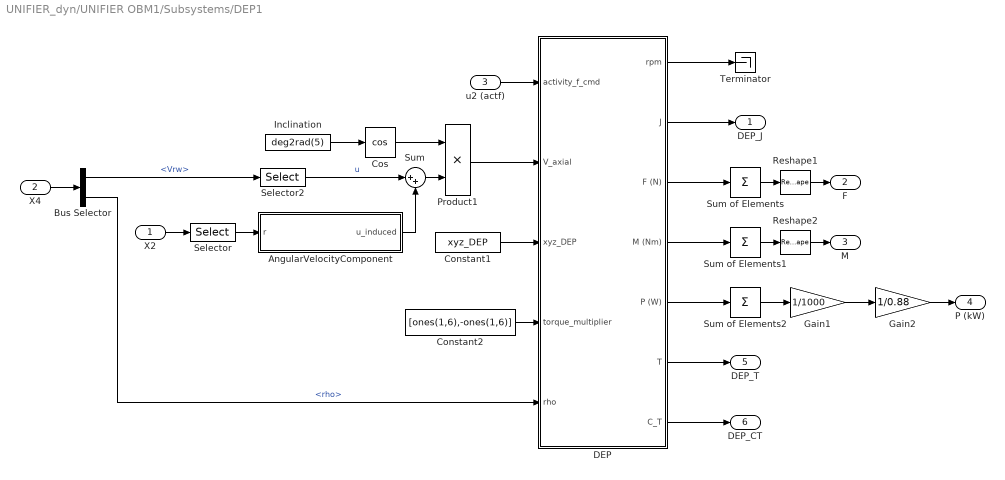
== system UNIFIER_dyn/UNIFIER OBM1/Subsystems/DEP1 ==
  X2 : Inport
  X4 : Inport  Port=2
  u2 (actf) : Inport  Port=3
  AngularVelocityComponent : Subsystem
  Bus Selector : BusSelector  OutputSignals=Vrw,rho
  Constant1 : Constant  Value=xyz_DEP
  Constant2 : Constant  Value=[ones(1,6),-ones(1,6)]
  Cos : Trigonometry  Operator=cos
  DEP : Subsystem  TreatAsAtomicUnit=on
  Gain1 : Gain  Gain=1/1000
  Gain2 : Gain  Gain=1/0.88
  Inclination : Constant  Value=deg2rad(5)
  Product1 : Product
  Reshape1 : Reshape
  Reshape2 : Reshape
  Selector : Selector  InputPortWidth=6  IndexOptions=Index vector (dialog)  Indices=6  OutputSizes=1
  Selector2 : Selector  InputPortWidth=3  IndexOptions=Index vector (dialog)  Indices=1  OutputSizes=1
  Sum : Sum  Inputs=|++
  Sum of Elements : Sum  Inputs=+  CollapseMode=Specified dimension  CollapseDim=2
  Sum of Elements1 : Sum  Inputs=+  CollapseMode=Specified dimension  CollapseDim=2
  Sum of Elements2 : Sum  Inputs=+  CollapseMode=Specified dimension
  Terminator : Terminator
  DEP_J : Outport
  F : Outport  Port=2
  M : Outport  Port=3
  P (kW) : Outport  Port=4
  DEP_T : Outport  Port=5
  DEP_CT : Outport  Port=6
  wires:
  DEP/1(rpm) -> Terminator/1
  AngularVelocityComponent/1(u_induced) -> Sum/2
  Selector/1 -> AngularVelocityComponent/1(r)
  Gain2/1 -> P (kW)/1
  Gain1/1 -> Gain2/1
  Sum/1 -> Product1/2
  Cos/1 -> Product1/1
  Inclination/1 -> Cos/1
  Selector2/1 -> Sum/1  "u"
  Sum of Elements2/1 -> Gain1/1
  DEP/5(P (W)) -> Sum of Elements2/1
  DEP/2(J) -> DEP_J/1
  Bus Selector/2 -> DEP/5(rho)  "<rho>"
  Constant2/1 -> DEP/4(torque_multiplier)
  Constant1/1 -> DEP/3(xyz_DEP)
  Reshape2/1 -> M/1
  Reshape1/1 -> F/1
  Sum of Elements1/1 -> Reshape2/1
  Sum of Elements/1 -> Reshape1/1
  DEP/4(M (Nm)) -> Sum of Elements1/1
  DEP/3(F (N)) -> Sum of Elements/1
  u2 (actf)/1 -> DEP/1(activity_f_cmd)
  Product1/1 -> DEP/2(V_axial)
  Bus Selector/1 -> Selector2/1  "<Vrw>"
  X4/1 -> Bus Selector/1
  X2/1 -> Selector/1
  DEP/6(T) -> DEP_T/1
  DEP/7(C_T) -> DEP_CT/1

== system UNIFIER_dyn/UNIFIER OBM1/Subsystems/Gravity ==
  X4 : Inport
  Bus Selector : BusSelector  OutputSignals=DCMbe
  Constant : Constant  Value=0
  Constant1 : Constant  Value=m
  Multiply : Gain  Gain=9.80665
  Mux : Mux  Inputs=3
  Product : Product  Multiplication=Matrix(*)
  F : Outport
  wires:
  Constant1/1 -> Multiply/1
  Mux/1 -> Product/2
  Constant/1 -> Mux/1, Mux/2
  Multiply/1 -> Mux/3
  X4/1 -> Bus Selector/1
  Bus Selector/1 -> Product/1  "<DCMbe>"
  Product/1 -> F/1  "F"

== system UNIFIER_dyn/UNIFIER OBM1/Subsystems/HTU ==
  u3 (actf) : Inport
  X4 : Inport  Port=2
  1-D Lookup Table1 : Lookup_n-D  NumberOfTableDimensions=1  BreakpointsForDimension1=[-0.5,1.5]  IndexSearchMethod=Linear search  BeginIndexSearchUsingPreviousIndexResult=on  Table=[-5000, 15000]  ExtrapMethod=Clip  InternalRulePriority=Speed  RndMeth=Simplest
  Bus Selector : BusSelector  OutputSignals=Vrw_mag_eas
  Constant : Constant  Value=0
  Gain : Gain  Gain=1/0.92
  Mux : Mux  Inputs=3
  Mux1 : Mux  Inputs=3
  PropAndMotor : Subsystem
  F (N) : Outport
  M (Nm) : Outport  Port=2
  P (kW) : Outport  Port=3
  wires:
  Gain/1 -> P (kW)/1
  u3 (actf)/1 -> 1-D Lookup Table1/1
  Bus Selector/1 -> PropAndMotor/1(Vrw_mag_eas)  "<Vrw_mag_eas>"
  1-D Lookup Table1/1 -> PropAndMotor/2(T_cmd (N))
  X4/1 -> Bus Selector/1
  PropAndMotor/1(P (kW)) -> Gain/1
  PropAndMotor/2(T (N)) -> Mux/1
  Mux/1 -> F (N)/1
  Constant/1 -> Mux/2, Mux/3, Mux1/1, Mux1/3, Mux1/2
  Mux1/1 -> M (Nm)/1

== system UNIFIER_dyn/UNIFIER OBM1/Aero/AlphaWIng/ComputeAlphaBetaV ==
  V_w_local : Inport
  Asin : Trigonometry  Operator=asin
  Atan : Trigonometry  Operator=atan
  Constant1 : Constant  Value=eps  OutDataTypeStr=single
  Demux : Demux  Outputs=3
  Divide : Product  Inputs=*/
  Divide1 : Product  Inputs=*/
  Dot Product : DotProduct  OutDataTypeStr=Inherit: Inherit via internal rule
  Square Root : Sqrt
  Sum2 : Sum  Inputs=|++
  alpha_nodes : Outport
  beta_nodes : Outport  Port=2
  V_nodes : Outport  Port=3
  wires:
  Atan/1 -> alpha_nodes/1
  Dot Product/1 -> Square Root/1
  Constant1/1 -> Sum2/2
  Asin/1 -> beta_nodes/1  "beta"
  Demux/3 -> Divide/1  "w"
  Divide/1 -> Atan/1
  Square Root/1 -> Divide1/2, V_nodes/1
  Sum2/1 -> Divide/2
  Demux/1 -> Sum2/1  "u"
  Divide1/1 -> Asin/1
  Demux/2 -> Divide1/1
  V_w_local/1 -> Demux/1, Dot Product/2, Dot Product/1

== system UNIFIER_dyn/UNIFIER OBM1/Aero/FinFuselageForces/Subsystem1 ==
  beta : Inport
  alpha : Inport  Port=2
  Constant : Constant  Value=0  OutDataTypeStr=single
  Interpolation Using Prelookup : Interpolation_n-D  Table=dp_FUSE_FIN.CD  InternalRulePriority=Speed  TableDataTypeStr=single
  Interpolation Using Prelookup1 : Interpolation_n-D  Table=dp_FUSE_FIN.CS  InternalRulePriority=Speed
  Interpolation Using Prelookup3 : Interpolation_n-D  Table=dp_FUSE_FIN.CMx  InternalRulePriority=Speed
  Interpolation Using Prelookup4 : Interpolation_n-D  Table=dp_FUSE_FIN.CMy  InternalRulePriority=Speed
  Interpolation Using Prelookup5 : Interpolation_n-D  Table=dp_FUSE_FIN.CMz  InternalRulePriority=Speed
  Subsystem : Subsystem
  Cd : Outport
  Cs : Outport  Port=2
  Cl : Outport  Port=3
  CMx : Outport  Port=4
  CMy : Outport  Port=5
  CMz : Outport  Port=6
  wires:
  Subsystem/2(Out2) -> Interpolation Using Prelookup5/2, Interpolation Using Prelookup4/2, Interpolation Using Prelookup3/2, Interpolation Using Prelookup1/2, Interpolation Using Prelookup/2
  Subsystem/1(Out1) -> Interpolation Using Prelookup5/1, Interpolation Using Prelookup4/1, Interpolation Using Prelookup3/1, Interpolation Using Prelookup1/1, Interpolation Using Prelookup/1
  Subsystem/4(Out4) -> Interpolation Using Prelookup5/4, Interpolation Using Prelookup4/4, Interpolation Using Prelookup3/4, Interpolation Using Prelookup1/4, Interpolation Using Prelookup/4
  Interpolation Using Prelookup1/1 -> Cs/1
  alpha/1 -> Subsystem/2(alpha)
  Interpolation Using Prelookup4/1 -> CMy/1
  Subsystem/3(Out3) -> Interpolation Using Prelookup5/3, Interpolation Using Prelookup4/3, Interpolation Using Prelookup3/3, Interpolation Using Prelookup1/3, Interpolation Using Prelookup/3
  beta/1 -> Subsystem/1(beta)
  Interpolation Using Prelookup5/1 -> CMz/1
  Constant/1 -> Cl/1
  Interpolation Using Prelookup/1 -> Cd/1
  Interpolation Using Prelookup3/1 -> CMx/1

== system UNIFIER_dyn/UNIFIER OBM1/Aero/InducedAngleOfAttack/preLook ==
  wing_flap_defl : Inport
  wing_alphas : Inport  Port=2
  wing_V_inf : Inport  Port=3
  wing_DEP_J : Inport  Port=4
  Constant8 : Constant  Value=0:15
  Prelookup : PreLookup  BreakpointsData=dp_VTAIL_INDUCED.flap_defl  IndexSearchMethod=Linear search  BeginIndexSearchUsingPreviousIndexResult=on  ExtrapMethod=Linear
  Prelookup1 : PreLookup  BreakpointsData=dp_VTAIL_INDUCED.V_infs  IndexSearchMethod=Linear search  BeginIndexSearchUsingPreviousIndexResult=on  ExtrapMethod=Linear
  Prelookup2 : PreLookup  BreakpointsData=dp_VTAIL_INDUCED.alphas  IndexSearchMethod=Linear search  BeginIndexSearchUsingPreviousIndexResult=on  ExtrapMethod=Linear
  Prelookup3 : PreLookup  BreakpointsData=dp_VTAIL_INDUCED.DEP_J  IndexSearchMethod=Linear search  BeginIndexSearchUsingPreviousIndexResult=on
  Out1 : Outport
  Out2 : Outport  Port=2
  Out8 : Outport  Port=3
  Out9 : Outport  Port=4
  Out3 : Outport  Port=5
  Out4 : Outport  Port=6
  Out6 : Outport  Port=7
  Out7 : Outport  Port=8
  Out5 : Outport  Port=9
  wires:
  Prelookup2/2 -> Out9/1
  Prelookup2/1 -> Out8/1
  Prelookup3/2 -> Out7/1
  Prelookup3/1 -> Out6/1
  wing_DEP_J/1 -> Prelookup3/1
  wing_alphas/1 -> Prelookup2/1
  wing_flap_defl/1 -> Prelookup/1
  Prelookup1/1 -> Out3/1
  wing_V_inf/1 -> Prelookup1/1
  Prelookup/2 -> Out2/1
  Prelookup1/2 -> Out4/1
  Constant8/1 -> Out5/1
  Prelookup/1 -> Out1/1

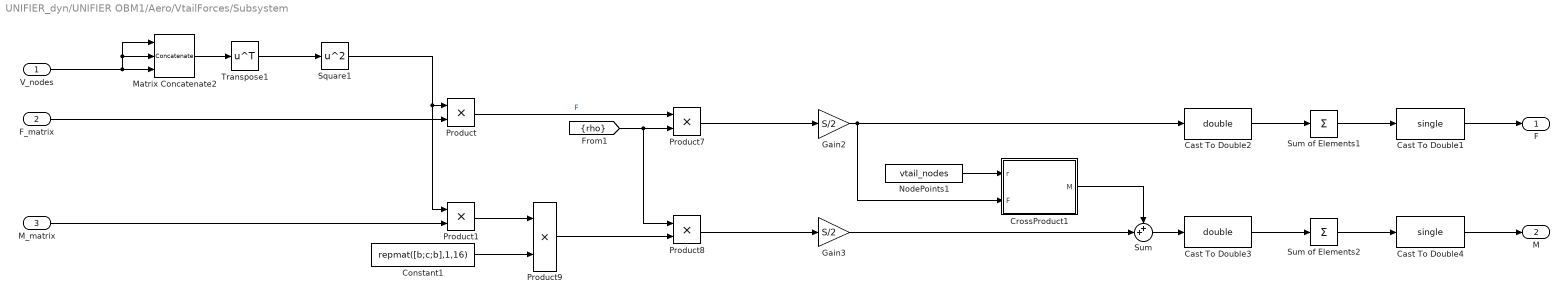
== system UNIFIER_dyn/UNIFIER OBM1/Aero/VtailForces/Subsystem ==
  V_nodes : Inport
  F_matrix : Inport  Port=2
  M_matrix : Inport  Port=3
  Cast To Double1 : DataTypeConversion  OutDataTypeStr=single  SaturateOnIntegerOverflow=off  RndMeth=Floor
  Cast To Double2 : DataTypeConversion  OutDataTypeStr=double  SaturateOnIntegerOverflow=off  RndMeth=Floor
  Cast To Double3 : DataTypeConversion  OutDataTypeStr=double  SaturateOnIntegerOverflow=off  RndMeth=Floor
  Cast To Double4 : DataTypeConversion  OutDataTypeStr=single  SaturateOnIntegerOverflow=off  RndMeth=Floor
  Constant1 : Constant  Value=repmat([b;c;b],1,16)  VectorParams1D=off  OutDataTypeStr=single
  CrossProduct1 : Subsystem  TreatAsAtomicUnit=on
  Gain2 : Gain  Gain=S/2
  Gain3 : Gain  Gain=S/2
  Matrix Concatenate2 : Concatenate  NumInputs=3  Mode=Multidimensional array  ConcatenateDimension=2
  NodePoints1 : Constant  Value=vtail_nodes
  Product{,1,7..9} (5 alike) : Product
  Square1 : Math  Operator=square
  Sum : Sum  Inputs=++|
  Sum of Elements1 : Sum  Inputs=+  CollapseMode=Specified dimension  CollapseDim=2
  Sum of Elements2 : Sum  Inputs=+  CollapseMode=Specified dimension  CollapseDim=2
  Transpose1 : Math  Operator=transpose
  F : Outport
  M : Outport  Port=2
  wires:
  Cast To Double4/1 -> M/1
  Cast To Double3/1 -> Sum of Elements2/1
  Cast To Double1/1 -> F/1
  Cast To Double2/1 -> Sum of Elements1/1
  V_nodes/1 -> Matrix Concatenate2/3, Matrix Concatenate2/2, Matrix Concatenate2/1
  F_matrix/1 -> Product/2
  CrossProduct1/1(M) -> Sum/1
  Product1/1 -> Product9/1
  M_matrix/1 -> Product1/2
  Constant1/1 -> Product9/2
  Product8/1 -> Gain3/1
  [rho] -> Product7/2, Product8/1
  NodePoints1/1 -> CrossProduct1/1(r)
  Product9/1 -> Product8/2
  Gain3/1 -> Sum/2
  Matrix Concatenate2/1 -> Transpose1/1
  Square1/1 -> Product/1, Product1/1
  Product7/1 -> Gain2/1
  Product/1 -> Product7/1  "F"
  Transpose1/1 -> Square1/1
  Sum of Elements1/1 -> Cast To Double1/1
  Sum of Elements2/1 -> Cast To Double4/1
  Gain2/1 -> Cast To Double2/1, CrossProduct1/2(F)
  Sum/1 -> Cast To Double3/1
